simulink model "manning_test_system_nonlinear"  (R2022b)
settings: Solver=VariableStepAuto  StartTime=0.0  StopTime=5*N  RelTol=1e-3
undefined symbols (not defined in the file): yd_ds, yu_ds
settings Model: Creator=chuan  LastModifiedBy=chuan

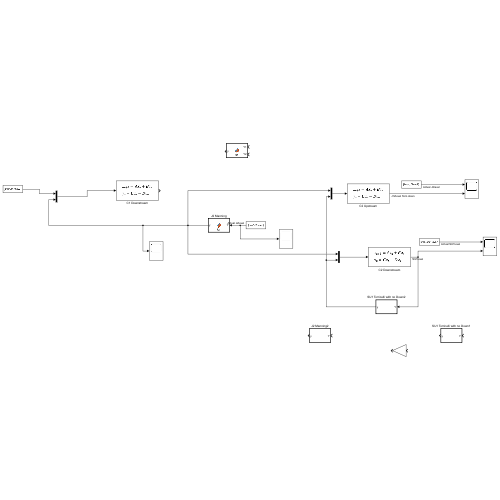
[thumbnail: Simulink's stored preview of the top-level diagram]
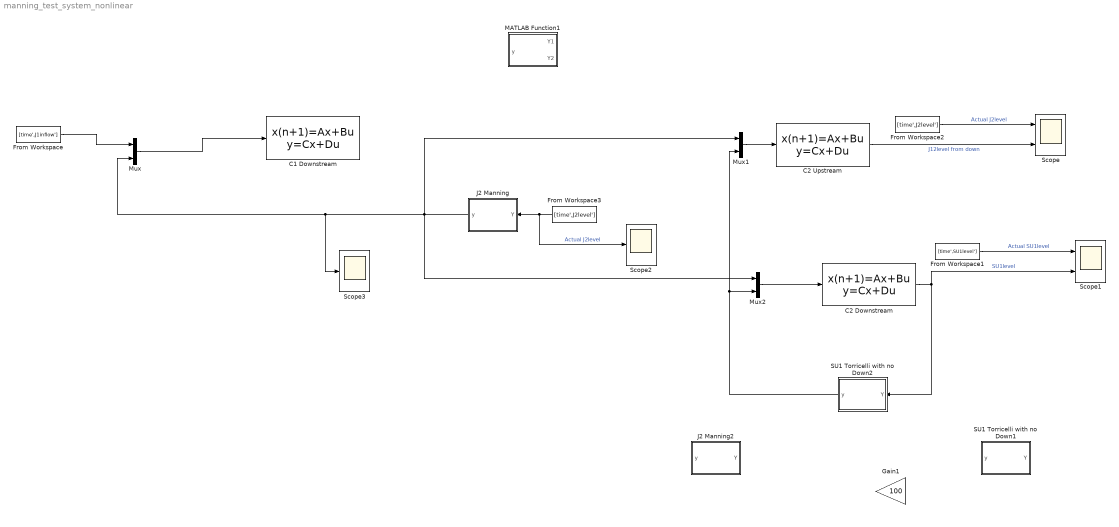
== system manning_test_system_nonlinear ==
  C1 Downstream : DiscreteStateSpace  A=yd_ds{1}.A  B=yd_ds{1}.B  C=yd_ds{1}.C  D=yd_ds{1}.D  SampleTime=yd_ds{1}.Ts
  C2 Downstream : DiscreteStateSpace  A=yd_ds{2}.A  B=yd_ds{2}.B  C=yd_ds{2}.C  D=yd_ds{2}.D  SampleTime=yd_ds{2}.Ts
  C2 Upstream : DiscreteStateSpace  A=yu_ds{2}.A  B=yu_ds{2}.B  C=yu_ds{2}.C  D=yu_ds{2}.D  SampleTime=yu_ds{2}.Ts
  From Workspace : FromWorkspace  VariableName=[time',J1inflow']
  From Workspace1 : FromWorkspace  VariableName=[time',SU1level']
  From Workspace2 : FromWorkspace  VariableName=[time',J2level']
  From Workspace3 : FromWorkspace  VariableName=[time',J2level']
  Gain1 : Gain  Gain=100
  J2 Manning : MATLAB Function  TreatAsAtomicUnit=on
  J2 Manning2 : MATLAB Function  TreatAsAtomicUnit=on
  MATLAB Function1 : MATLAB Function  TreatAsAtomicUnit=on
  Mux : Mux  Inputs=2
  Mux1 : Mux  Inputs=2
  Mux2 : Mux  Inputs=2
  SU1 Torricelli with no Down1 : MATLAB Function  TreatAsAtomicUnit=on
  SU1 Torricelli with no Down2 : MATLAB Function  TreatAsAtomicUnit=on
  Scope : Scope  NumInputPorts=2
  Scope1 : Scope  NumInputPorts=2
  Scope2 : Scope
  Scope3 : Scope
  wires:
  Mux/1 -> C1 Downstream/1
  From Workspace/1 -> Mux/1
  From Workspace2/1 -> Scope/1  "Actual J2level"
  Mux1/1 -> C2 Upstream/1
  SU1 Torricelli with no Down2/1(y) -> Mux2/2, Mux1/2
  Mux2/1 -> C2 Downstream/1
  C2 Downstream/1 -> SU1 Torricelli with no Down2/1(Y), Scope1/2  "SU1level"
  From Workspace1/1 -> Scope1/1  "Actual SU1level"
  J2 Manning/1(y) -> Mux2/1, Mux1/1, Scope3/1, Mux/2
  C2 Upstream/1 -> Scope/2  "J12level from down"
  From Workspace3/1 -> Scope2/1, J2 Manning/1(Y)  "Actual J2level"

== matlab function manning_test_system_nonlinear/J2 Manning2 ==
  data: Y input; y output
function y = fcn(Y)
n = 0.015;
Sb = 0.0005;
B=8;
m = 1.5;

Y = max(Y,0);

y = (1/n)*(B*Y + m*Y.^2)*((B*Y + m*Y.^2)/(B + 2.*Y.*sqrt(1+m^2))).^(2/3) .* sqrt(Sb);

== matlab function manning_test_system_nonlinear/J2 Manning ==
  data: Y input; y output
function y = fcn(Y)
n = 0.015;
Sb = 0.0005;
B=8;
m = 1.5;

Y = max(Y,0);

y = (1/n)*(B*Y + m*Y.^2)*((B*Y + m*Y.^2)/(B + 2.*Y.*sqrt(1+m^2))).^(2/3) .* sqrt(Sb);

== matlab function manning_test_system_nonlinear/SU1 Torricelli with no Down1 ==
  data: Y input; y output
function y = fcn(Y)
Cd = 0.65;
A0 = 4;
g = 9.81;
Z0 = 9;
Yfull = 2;
H_star = Z0 + Yfull;

Y = max(Y,0);
H1 = Y + Z0;

if H1 >= H_star
    He = H1 - (Z0 + Yfull/2);
    y = Cd*A0*sqrt(2*g*He);
else
    CwL = (Cd*A0*sqrt(g))/(Yfull);
    y = CwL*(H1-Z0)^(1.5);
end

== matlab function manning_test_system_nonlinear/MATLAB Function1 ==
  data: Y1 input; y output; Y2 input
function y = fcn(Y1,Y2)
Cd = 0.65;
A0 = 36;
g = 9.81;
Z0 = 5.6;
Yfull = 6;
H_star = Z0 + Yfull;

Y1 = max(Y1,0);
Y2 = max(Y2,0);
H1 = Y1 + Z0;
H2 = Y2 + Z0;

if H1 >= H_star
    if H2 <= Z0 + Yfull/2
        He = H1 - (Z0 + Yfull/2);
    else
        He = H1-H2;
    end

    if He >= 0
        y = Cd*A0*sqrt(2*g*He);
    else
        y = -Cd*A0*sqrt(2*g*-He);
    end
else
    CwL = (Cd*A0*sqrt(g))/(Yfull);
    y = CwL*(H1-Z0)^(1.5);
end

== matlab function manning_test_system_nonlinear/SU1 Torricelli with no Down2 ==
  data: Y input; y output
function y = fcn(Y)
Cd = 0.65;
A0 = 4;
g = 9.81;
Z0 = 9;
Yfull = 2;
H_star = Z0 + Yfull;

Y = max(Y,0);
H1 = Y + Z0;

if H1 >= H_star
    He = H1 - (Z0 + Yfull/2);
    y = Cd*A0*sqrt(2*g*He);
else
    CwL = (Cd*A0*sqrt(g))/(Yfull);
    y = CwL*(H1-Z0)^(1.5);
end
